simulink model "reconstructed_model_layout2_left_to_right_signal_flow"  (R2024a)
settings: Solver=VariableStepAuto  StartTime=0.0  StopTime=10.0  RelTol=1e-3
settings Model: Creator=jacky  LastModifiedBy=jacky

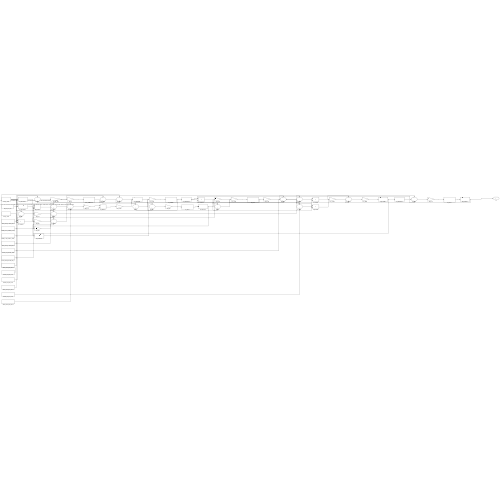
[thumbnail: Simulink's stored preview of the top-level diagram]
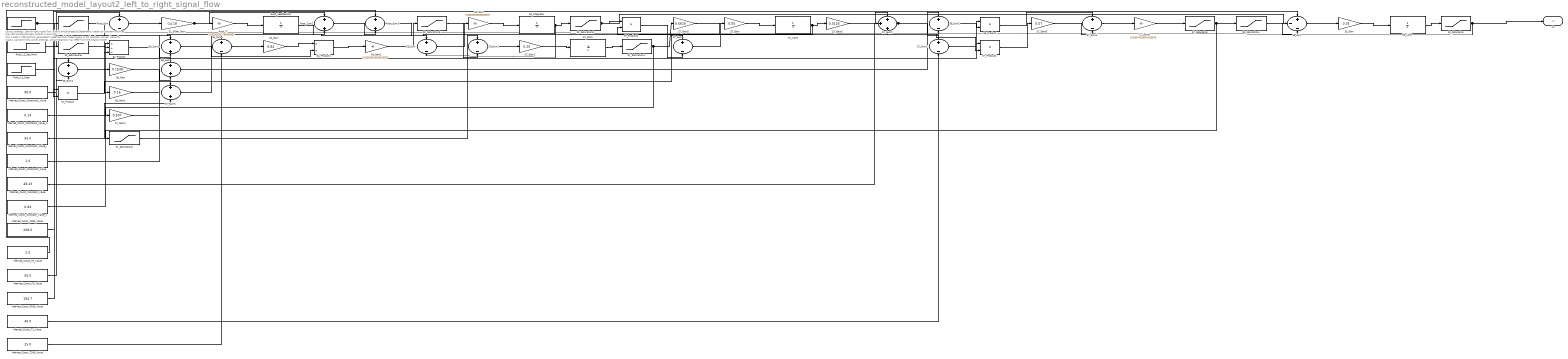
== system reconstructed_model_layout2_left_to_right_signal_flow ==
  note: Layout strategy: Left-to-right signal flow. Blocks are arranged by dependency depth so upstream sources stay left and downstream outputs move right.
  note: This model is inferred from generated C code. Simulink Coder output is not lossless; names, hierarchy, masks, sample times, solver settings, and annotations may differ from the original model.
  Root_F1_Step : Step  Time=200.0  Before=10.0  After=10.0  SampleTime=0
  Root_FeedbackInt : Integrator  InitialCondition=0.0
  Root_L2_Set_Point : Step  Time=200.0  Before=1.0  After=1.0  SampleTime=0
  Root_Sum : Sum  Inputs=+-
  Root_Sum1 : Sum
  Root_Sum2 : Sum
  Root_Ti : Gain  Gain=0.052826201796090863
  Root_X1_Step : Step  Time=200.0  Before=5.0  After=35.0  SampleTime=0
  S1_Slider_Gain : Gain  Gain=-14.18
  S2_Saturation : Saturate  UpperLimit=2.0  LowerLimit=0.0
  S2_Saturation2 : Saturate  UpperLimit=400.0  LowerLimit=0.0
  S2_Saturation3 : Saturate  UpperLimit=4.0  LowerLimit=0.0
  S2_Saturation4 : Saturate  UpperLimit=16.0  LowerLimit=0.0
  S2_Saturation5 : Saturate  UpperLimit=16.0  LowerLimit=0.0
  S2_Saturation6 : Saturate  UpperLimit=416.0  LowerLimit=0.0
  S3_Gain : Gain  Gain=0.83333333333333337
  S3_Integrator : Integrator  InitialCondition=0.0
  S3_Sum : Sum  Inputs=+-
  S4_Gain : Gain  Gain=6.84
  S4_Gain1 : Gain  Gain=0.025974025974025976
  S4_Product : Product  Inputs=*//
  S4_Product1 : Product  Inputs=*/
  S4_Sum : Sum  Inputs=+-
  S4_Sum1 : Sum
  S5_Gain : Gain  Gain=0.05
  S5_L2Int : Integrator  InitialCondition=1.0
  S5_Sum : Sum  Inputs=+--
  S6_Gain : Gain  Gain=0.1538
  S6_Gain1 : Gain  Gain=0.16
  S6_Product : Product  Inputs=**
  S6_Sum : Sum
  S6_Sum1 : Sum
  S6_Sum2 : Sum  Inputs=+-
  S7_Gain : Gain  Gain=0.05
  S7_Gain1 : Gain  Gain=0.25
  S7_Gain2 : Gain  Gain=0.5616
  S7_Gain3 : Gain  Gain=0.3126
  S7_Gain4 : Gain  Gain=0.507
  S7_Gain5 : Gain  Gain=0.07
  S7_Gain6 : Gain  Gain=0.025974025974025976
  S7_P2Int : Integrator  InitialCondition=50.5
  S7_Product : Product  Inputs=**
  S7_Product1 : Product  Inputs=**
  S7_Product2 : Product  Inputs=**
  S7_Saturation : Saturate  UpperLimit=16.0  LowerLimit=0.0
  S7_Saturation1 : Saturate  UpperLimit=100.0  LowerLimit=0.0
  S7_Saturation2 : Saturate  UpperLimit=16.0  LowerLimit=0.0
  S7_Sum{,1,4..5} (4 alike) : Sum  Inputs=+-
  S7_Sum2 : Sum  Inputs=+++
  S7_Sum3 : Sum
  S7_X2Int : Integrator  InitialCondition=25.0
  inferred_Const_Constant1_Value : Constant  Value=90.0
  inferred_Const_Constant1_Value_h : Constant  Value=0.14
  inferred_Const_Constant1_Value_i : Constant  Value=55.0
  inferred_Const_Constant2_Value : Constant  Value=1.0
  inferred_Const_Constant_Value : Constant  Value=48.43
  inferred_Const_Constant_Value_c : Constant  Value=6.84
  inferred_Const_F200_Value : Constant  Value=208.0
  inferred_Const_F2_Value : Constant  Value=2.0
  inferred_Const_F3_Value : Constant  Value=50.0
  inferred_Const_P100_Value : Constant  Value=194.7
  inferred_Const_T1_Value : Constant  Value=40.0
  inferred_Const_T200_Value : Constant  Value=25.0
  L2 : Outport
  wires:
  S2_Saturation/1 -> L2/1, Root_Sum/2
  Root_Ti/1 -> Root_FeedbackInt/1
  Root_L2_Set_Point/1 -> Root_Sum/1
  inferred_Const_F2_Value/1 -> Root_Sum1/1
  Root_Sum2/1 -> Root_Sum1/2
  S1_Slider_Gain/1 -> Root_Sum2/1, Root_Ti/1
  Root_FeedbackInt/1 -> Root_Sum2/2
  Root_Sum/1 -> S1_Slider_Gain/1
  S5_L2Int/1 -> S2_Saturation/1
  inferred_Const_P100_Value/1 -> S2_Saturation2/1
  S3_Integrator/1 -> S2_Saturation3/1, S3_Sum/2
  S7_Saturation/1 -> S2_Saturation4/1, S7_Saturation2/1
  S4_Gain1/1 -> S2_Saturation5/1
  inferred_Const_F200_Value/1 -> S2_Saturation6/1
  S3_Sum/1 -> S3_Gain/1
  S3_Gain/1 -> S3_Integrator/1
  Root_Sum1/1 -> S3_Sum/1
  S4_Sum/1 -> S4_Gain/1
  S4_Product1/1 -> S4_Gain1/1
  inferred_Const_Constant_Value_c/1 -> S4_Product/1
  inferred_Const_Constant1_Value_h/1 -> S4_Product/2
  S2_Saturation6/1 -> S4_Product/3
  S4_Gain/1 -> S4_Product1/1
  S4_Sum1/1 -> S4_Product1/2
  S7_Sum3/1 -> S4_Sum/1
  inferred_Const_T200_Value/1 -> S4_Sum/2
  inferred_Const_Constant2_Value/1 -> S4_Sum1/1
  S4_Product/1 -> S4_Sum1/2
  S5_Sum/1 -> S5_Gain/1
  S5_Gain/1 -> S5_L2Int/1
  Root_F1_Step/1 -> S5_Sum/1, S6_Sum1/1, S7_Product/1, S7_Product2/2
  S2_Saturation3/1 -> S5_Sum/2, S7_Product1/1
  S2_Saturation4/1 -> S5_Sum/3
  S2_Saturation2/1 -> S6_Gain/1
  S6_Sum1/1 -> S6_Gain1/1
  S6_Gain1/1 -> S6_Product/1
  S6_Sum2/1 -> S6_Product/2
  inferred_Const_Constant1_Value/1 -> S6_Sum/1
  S6_Gain/1 -> S6_Sum/2
  inferred_Const_F3_Value/1 -> S6_Sum1/2
  S6_Sum/1 -> S6_Sum2/1
  S7_Sum2/1 -> S6_Sum2/2, S7_Sum5/1
  S7_Sum/1 -> S7_Gain/1
  S7_Sum1/1 -> S7_Gain1/1
  S7_Saturation1/1 -> S7_Gain2/1, S7_Gain4/1
  S7_X2Int/1 -> S7_Gain3/1, S7_Product1/2
  S7_Product2/1 -> S7_Gain5/1
  S7_Sum4/1 -> S7_Gain6/1
  S7_Gain1/1 -> S7_P2Int/1
  Root_X1_Step/1 -> S7_Product/2
  S7_Sum5/1 -> S7_Product2/1
  S7_Gain6/1 -> S7_Saturation/1
  S7_P2Int/1 -> S7_Saturation1/1
  S7_Product/1 -> S7_Sum/1
  S7_Product1/1 -> S7_Sum/2
  S7_Saturation2/1 -> S7_Sum1/1
  S2_Saturation5/1 -> S7_Sum1/2
  S7_Gain3/1 -> S7_Sum2/1
  inferred_Const_Constant_Value/1 -> S7_Sum2/2
  S7_Gain2/1 -> S7_Sum2/3
  S7_Gain4/1 -> S7_Sum3/1
  inferred_Const_Constant1_Value_i/1 -> S7_Sum3/2
  S6_Product/1 -> S7_Sum4/1
  S7_Gain5/1 -> S7_Sum4/2
  inferred_Const_T1_Value/1 -> S7_Sum5/2
  S7_Gain/1 -> S7_X2Int/1
